simulink model "simulin10_1"  (R2025b)
settings: Solver=ode45  StartTime=0.0  StopTime=150.0  MaxStep=0.05  RelTol=1e-3
settings Model: Creator=mizula  LastModifiedBy=mizula

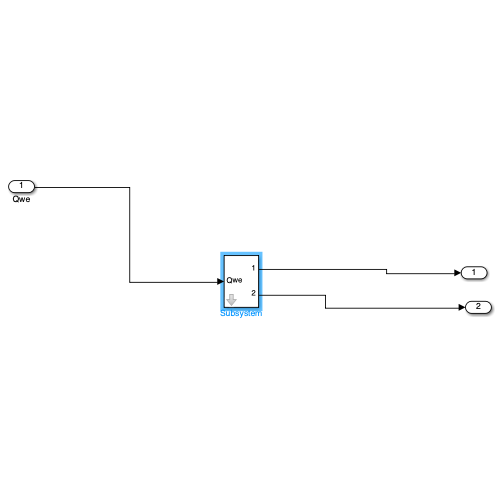
[thumbnail: Simulink's stored preview of the top-level diagram]
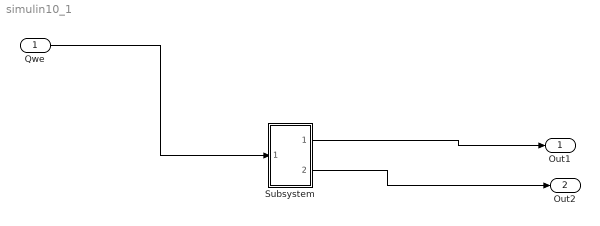
== system simulin10_1 ==
  Qwe : Inport
  Subsystem : Subsystem  mask{S1=1, S2=2, Swy1=0.2, Swy2=0.2, fi1=1, fi2=1, g=9.81, h1=4, h2=2}
  Out1 : Outport
  Out2 : Outport  Port=2
  wires:
  Qwe/1 -> Subsystem/1(Qwe)
  Subsystem/1(Out1) -> Out1/1
  Subsystem/2(Out2) -> Out2/1

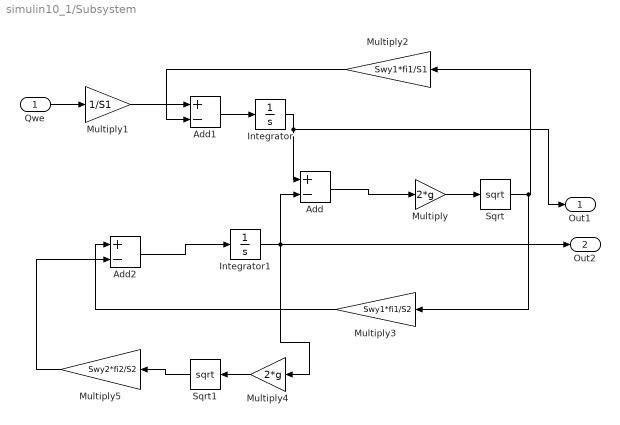
== system simulin10_1/Subsystem ==
  Qwe : Inport
  Add : Sum  Inputs=+-
  Add1 : Sum  Inputs=+-
  Add2 : Sum  Inputs=+-
  Integrator : Integrator  InitialCondition=h1
  Integrator1 : Integrator  InitialCondition=h2
  Multiply : Gain  Gain=2*g
  Multiply1 : Gain  Gain=1/S1
  Multiply2 : Gain  Gain=Swy1*fi1/S1
  Multiply3 : Gain  Gain=Swy1*fi1/S2
  Multiply4 : Gain  Gain=2*g
  Multiply5 : Gain  Gain=Swy2*fi2/S2
  Sqrt : Sqrt
  Sqrt1 : Sqrt
  Out1 : Outport
  Out2 : Outport  Port=2
  wires:
  Multiply3/1 -> Add2/1
  Multiply2/1 -> Add1/2
  Add2/1 -> Integrator1/1
  Sqrt1/1 -> Multiply5/1
  Add1/1 -> Integrator/1
  Multiply1/1 -> Add1/1
  Sqrt/1 -> Multiply3/1, Multiply2/1
  Multiply/1 -> Sqrt/1
  Multiply5/1 -> Add2/2
  Multiply4/1 -> Sqrt1/1
  Qwe/1 -> Multiply1/1
  Integrator/1 -> Out1/1, Add/1
  Add/1 -> Multiply/1
  Integrator1/1 -> Out2/1, Multiply4/1, Add/2
